simulink model "walkingRobotRL3D"  (R2020b)
settings: Solver=ode23t  StartTime=0.0  StopTime=Tf  RelTol=1e-2  EnableMultiTasking=on
PreLoadFcn:
  | robotParametersRL
undefined symbols (not defined in the file): agent, ankleD_pitch_jointMAX, ankleD_pitch_jointMIN, ankleD_roll_jointMAX, ankleD_roll_jointMIN, ankleI_pitch_jointMAX, ankleI_pitch_jointMIN, ankleI_roll_jointMAX, ankleI_roll_jointMIN, getSampleTime, height_plane, hipD_pitch_jointMAX, hipD_pitch_jointMIN, hipD_roll_jointMAX, hipD_roll_jointMIN, hipI_pitch_jointMAX, hipI_pitch_jointMIN, hipI_roll_jointMAX, hipI_roll_jointMIN, init_angs_L, init_angs_R, init_height, joint_damping, joint_limit_damping, joint_limit_stiffness, joint_stiffness, kneeD_jointMAX, kneeD_jointMIN, kneeI_jointMAX, kneeI_jointMIN, lower_leg_I0, lower_leg_length, lower_leg_mass, lower_leg_x, lower_leg_y, muscle_nominal_length, p10_ankleD_roll, plane_x, plane_y, regulator_type, tau, Tf, torso_height, torso_length, torso_offset_x, torso_offset_z, torso_width, torso_x, torso_y, torso_z, Ts, upper_leg_I0, upper_leg_length, upper_leg_mass, upper_leg_x, upper_leg_y, v10_ankleD_pitch, v10_ankleD_roll, v10_ankleI_pitch, v10_ankleI_roll ... (+41)
libraries: sm_lib x222, simulink x183, nesl_utility x130, walkingRobotUtils x69, rllib x2
(part 19 of 24)

== matlab function walkingRobotRL3D/Walking Robot/DYNAMIC MODEL OF PAM FOR LEFT LEG/Dynamic Model Antagonisitic PAM2/Proportional Regulator (Muscles 1) ==
  data: V1 input; reg_type input; p1 output
% Author: Eduardo Reyero Ibáñez
% Descrition: In this file it will be implemented the required input for the PAM
function p1  = propReg(V1,reg_type)
%% Proportional pressure regulators VPPM
%Range of Voltage
minVoltage = 0;
maxVoltage = 7.98; % This voltage provide 8 bar of pressure with regulator type 1
p1 = zeros(1,1);
%Select regulartor type
%reg_type = 1; % This will be given by the call of the function
%Limit the voltage
for i=1:length(p1)
if V1(i) >= maxVoltage 
    V1(i) = maxVoltage;
end
end
if reg_type == 1
    f_prop = @(V) 0.99*V+0.1;
    for i=1:length(p1)
    p1(i) = f_prop(V1(i));
    end
elseif reg_type == 2
    f_prop = @(V) 0.594*V+0.06;
    for i=1:length(p1)
    p1(i) = f_prop(V1(i));
    end
else
    f_prop = @(V) 0.198*V+0.02;
    for i=1:length(p1)
    p1(i) = f_prop(V1(i));
    end
end

% figure
% fplot(p1)
% xlim([0 10])
% ylim([0 10])
end

== matlab function walkingRobotRL3D/Walking Robot/DYNAMIC MODEL OF PAM FOR LEFT LEG/Dynamic Model Antagonisitic PAM2/Proportional Regulator (Muscles 2) ==
  data: V1 input; reg_type input; p1 output
% Author: Eduardo Reyero Ibáñez
% Descrition: In this file it will be implemented the required input for the PAM
function p1  = propReg(V1,reg_type)
%% Proportional pressure regulators VPPM
%Range of Voltage
minVoltage = 0;
maxVoltage = 7.98; % This voltage provide 8 bar of pressure with regulator type 1
p1 = zeros(1,1);
%Select regulartor type
%reg_type = 1; % This will be given by the call of the function
%Limit the voltage
for i=1:length(p1)
if V1(i) >= maxVoltage 
    V1(i) = maxVoltage;
end
end
if reg_type == 1
    f_prop = @(V) 0.99*V+0.1;
    for i=1:length(p1)
    p1(i) = f_prop(V1(i));
    end
elseif reg_type == 2
    f_prop = @(V) 0.594*V+0.06;
    for i=1:length(p1)
    p1(i) = f_prop(V1(i));
    end
else
    f_prop = @(V) 0.198*V+0.02;
    for i=1:length(p1)
    p1(i) = f_prop(V1(i));
    end
end

% figure
% fplot(p1)
% xlim([0 10])
% ylim([0 10])
end

== matlab function walkingRobotRL3D/Walking Robot/DYNAMIC MODEL OF PAM FOR LEFT LEG/Dynamic Model Antagonisitic PAM2/Spring and damping model/S(P),D(P) ==
  data: P1 input; S1 output; P2 input; D1 output; S2 output; D2 output
function [S1,D1,S2,D2] = getSpringDampingCoeff(P1,P2)
tau = 0.6;
% Spring and damping coeff for muscle 1
if P1>=0 && P1<=1
    S1 = 400;
    D1 = tau*S1;
elseif P1>1 && P1<=2
    S1 = 500;
    D1 = tau*S1;
elseif P1>2 && P1<=3
    S1 = 1100;
    D1 = tau*S1;
elseif P1>3 && P1<=4
    S1 = 1500;
    D1 = tau*S1;
elseif P1>4 && P1<=5
    S1 = 2000;
    D1 = tau*S1;
elseif P1>5 && P1<=6
    S1 = 2900;
    D1 = tau*S1;
elseif P1>6 && P1<=7
    S1 = 3800;
    D1 = tau*S1;
elseif P1>7 && P1<=8.5
    S1 = 5000;
    D1 = tau*S1;
else %Never will enter here
    S1 = 800;
    D1 = tau*S1;  
end

% Spring and damping coeff for muscle 1
if P2>=0 && P2<=1
    S2 = 400;
    D2 = tau*S2;
elseif P2>1 && P2<=2
    S2 = 500;
    D2 = tau*S2;
elseif P2>2 && P2<=3
    S2 = 1100;
    D2 = tau*S2;
elseif P2>3 && P2<=4
    S2 = 1500;
    D2 = tau*S2;
elseif P2>4 && P2<=5
    S2 = 2000;
    D2 = tau*S2;
elseif P2>5 && P2<=6
    S2 = 2900;
    D2 = tau*S2;
elseif P2>6 && P2<=7
    S2 = 3800;
    D2 = tau*S2;
elseif P2>7 && P2<=8.5
    S2 = 5000;
    D2 = tau*S2;
else %Never will enter here
    S2 = 800;
    D2 = tau*S2;  
end

end

== matlab function walkingRobotRL3D/Walking Robot/DYNAMIC MODEL OF PAM FOR LEFT LEG/Dynamic Model Antagonisitic PAM3/F(x,P) mode (Muscles 1) ==
  data: P1 input; F1 output; x_muscle1 input
%Author: Eduardo Reyero Ibáñez
%Note: F(x) curves for different pressures are limited by recommended
%limitation of 20% in contraction percentage for the used PAM actuator
%(L = 260mm D=20mm)
function F1 = FxPmodel(P1,x_muscle1)
%Input: P comming from proporcional controller  is in bar. Its 6x1 vector
% x_muscle (in % contraction)
%Output:F according to P input and and x value of half of the maximun
%permissible stroke
%Importing 2 variable F(x,P) model
curve = @(x,P)  -0.002697-93.8*x+2.917*P+13.05*x^2-0.04264*x*P-0.001793*P^2-0.9395*x^3-0.001597*x^2*P-0.0001142*x*P^2+4.694e-06*P^3+0.03335*x^4+6.106e-06*x^3*P+2.699e-06*x^2*P^2+1.25e-07*x*P^3-5.675e-09*P^4-0.0004611*x^5+9.334e-07*x^4*P-1.221e-08*x^3*P^2-1.463e-09*x^2*P^3-4.929e-11*x*P^4+2.492e-12*P^5;
%Defining F and x vectors for the 6 actuators
F1 = zeros(length(P1),1); %6x1
x1 = zeros(length(P1),1); %6x1
% Transform P from bar to Kpa
P1 = 100*P1;

for i=1:length(P1)
% Obtaining the stroke
x1(i) = x_muscle1(i); 
% Obtaining the applied force
F1(i) = curve(x1(i),P1(i)); 
if F1(i)<0
    F1(i) = 0;
end
end
end

== matlab function walkingRobotRL3D/Walking Robot/DYNAMIC MODEL OF PAM FOR LEFT LEG/Dynamic Model Antagonisitic PAM3/F(x,P) mode (Muscles 1)1 ==
  data: P2 input; F2 output; x_muscle2 input
%Author: Eduardo Reyero Ibáñez
%Note: F(x) curves for different pressures are limited by recommended
%limitation of 20% in contraction percentage for the used PAM actuator
%(L = 260mm D=20mm)
function F2 = FxPmodel(P2,x_muscle2)
%Input: P comming from proporcional controller  is in bar. Its 6x1 vector
% x_muscle (in % contraction)
%Output:F according to P input and and x value of half of the maximun
%permissible stroke
%Importing 2 variable F(x,P) model
curve = @(x,P)  -0.002697-93.8*x+2.917*P+13.05*x^2-0.04264*x*P-0.001793*P^2-0.9395*x^3-0.001597*x^2*P-0.0001142*x*P^2+4.694e-06*P^3+0.03335*x^4+6.106e-06*x^3*P+2.699e-06*x^2*P^2+1.25e-07*x*P^3-5.675e-09*P^4-0.0004611*x^5+9.334e-07*x^4*P-1.221e-08*x^3*P^2-1.463e-09*x^2*P^3-4.929e-11*x*P^4+2.492e-12*P^5;
%Defining F and x vectors for the 6 actuators
F2 = zeros(length(P2),1); %6x1
x2 = zeros(length(P2),1); %6x1
% Transform P from bar to Kpa
P2 = 100*P2;

for i=1:length(P2)
% Obtaining the stroke
x2(i) = x_muscle2(i); 
% Obtaining the applied force
F2(i) = curve(x2(i),P2(i));
if F2(i)<0
    F2(i) = 0;
end
end
end

== matlab function walkingRobotRL3D/Walking Robot1/Dynamic model of antagonistic PAM actuators/F(x,P) mode (Muscles 1) ==
  data: P1 input; F1 output; x_muscle1 input
%Author: Eduardo Reyero Ibáñez
%Note: F(x) curves for different pressures are limited by recommended
%limitation of 20% in contraction percentage for the used PAM actuator
%(L = 260mm D=20mm)
function F1 = FxPmodel(P1,x_muscle1)
%Input: P comming from proporcional controller  is in bar. Its 6x1 vector
% x_muscle (in % contraction)
%Output:F according to P input and and x value of half of the maximun
%permissible stroke
%Importing 2 variable F(x,P) model
curve = @(x,P)  -0.002697-93.8*x+2.917*P+13.05*x^2-0.04264*x*P-0.001793*P^2-0.9395*x^3-0.001597*x^2*P-0.0001142*x*P^2+4.694e-06*P^3+0.03335*x^4+6.106e-06*x^3*P+2.699e-06*x^2*P^2+1.25e-07*x*P^3-5.675e-09*P^4-0.0004611*x^5+9.334e-07*x^4*P-1.221e-08*x^3*P^2-1.463e-09*x^2*P^3-4.929e-11*x*P^4+2.492e-12*P^5;
%Defining F and x vectors for the 6 actuators
F1 = zeros(length(P1),1); %6x1
x1 = zeros(length(P1),1); %6x1
% Transform P from bar to Kpa
P1 = 100*P1;

for i=1:length(P1)
% Obtaining the stroke
x1(i) = x_muscle1(i); 
% Obtaining the applied force
F1(i) = curve(x1(i),P1(i)); 
end
end

== matlab function walkingRobotRL3D/Walking Robot/DYNAMIC MODEL OF PAM FOR LEFT LEG/Dynamic Model Antagonisitic PAM3/Proportional Regulator (Muscles 1) ==
  data: V1 input; reg_type input; p1 output
% Author: Eduardo Reyero Ibáñez
% Descrition: In this file it will be implemented the required input for the PAM
function p1  = propReg(V1,reg_type)
%% Proportional pressure regulators VPPM
%Range of Voltage
minVoltage = 0;
maxVoltage = 7.98; % This voltage provide 8 bar of pressure with regulator type 1
p1 = zeros(1,1);
%Select regulartor type
%reg_type = 1; % This will be given by the call of the function
%Limit the voltage
for i=1:length(p1)
if V1(i) >= maxVoltage 
    V1(i) = maxVoltage;
end
end
if reg_type == 1
    f_prop = @(V) 0.99*V+0.1;
    for i=1:length(p1)
    p1(i) = f_prop(V1(i));
    end
elseif reg_type == 2
    f_prop = @(V) 0.594*V+0.06;
    for i=1:length(p1)
    p1(i) = f_prop(V1(i));
    end
else
    f_prop = @(V) 0.198*V+0.02;
    for i=1:length(p1)
    p1(i) = f_prop(V1(i));
    end
end

% figure
% fplot(p1)
% xlim([0 10])
% ylim([0 10])
end

== matlab function walkingRobotRL3D/Walking Robot/DYNAMIC MODEL OF PAM FOR LEFT LEG/Dynamic Model Antagonisitic PAM3/Proportional Regulator (Muscles 2) ==
  data: V1 input; reg_type input; p1 output
% Author: Eduardo Reyero Ibáñez
% Descrition: In this file it will be implemented the required input for the PAM
function p1  = propReg(V1,reg_type)
%% Proportional pressure regulators VPPM
%Range of Voltage
minVoltage = 0;
maxVoltage = 7.98; % This voltage provide 8 bar of pressure with regulator type 1
p1 = zeros(1,1);
%Select regulartor type
%reg_type = 1; % This will be given by the call of the function
%Limit the voltage
for i=1:length(p1)
if V1(i) >= maxVoltage 
    V1(i) = maxVoltage;
end
end
if reg_type == 1
    f_prop = @(V) 0.99*V+0.1;
    for i=1:length(p1)
    p1(i) = f_prop(V1(i));
    end
elseif reg_type == 2
    f_prop = @(V) 0.594*V+0.06;
    for i=1:length(p1)
    p1(i) = f_prop(V1(i));
    end
else
    f_prop = @(V) 0.198*V+0.02;
    for i=1:length(p1)
    p1(i) = f_prop(V1(i));
    end
end

% figure
% fplot(p1)
% xlim([0 10])
% ylim([0 10])
end

== matlab function walkingRobotRL3D/Walking Robot/DYNAMIC MODEL OF PAM FOR LEFT LEG/Dynamic Model Antagonisitic PAM3/Spring and damping model/S(P),D(P) ==
  data: P1 input; S1 output; P2 input; D1 output; S2 output; D2 output
function [S1,D1,S2,D2] = getSpringDampingCoeff(P1,P2)
tau = 0.6;
% Spring and damping coeff for muscle 1
if P1>=0 && P1<=1
    S1 = 400;
    D1 = tau*S1;
elseif P1>1 && P1<=2
    S1 = 500;
    D1 = tau*S1;
elseif P1>2 && P1<=3
    S1 = 1100;
    D1 = tau*S1;
elseif P1>3 && P1<=4
    S1 = 1500;
    D1 = tau*S1;
elseif P1>4 && P1<=5
    S1 = 2000;
    D1 = tau*S1;
elseif P1>5 && P1<=6
    S1 = 2900;
    D1 = tau*S1;
elseif P1>6 && P1<=7
    S1 = 3800;
    D1 = tau*S1;
elseif P1>7 && P1<=8.5
    S1 = 5000;
    D1 = tau*S1;
else %Never will enter here
    S1 = 800;
    D1 = tau*S1;  
end

% Spring and damping coeff for muscle 1
if P2>=0 && P2<=1
    S2 = 400;
    D2 = tau*S2;
elseif P2>1 && P2<=2
    S2 = 500;
    D2 = tau*S2;
elseif P2>2 && P2<=3
    S2 = 1100;
    D2 = tau*S2;
elseif P2>3 && P2<=4
    S2 = 1500;
    D2 = tau*S2;
elseif P2>4 && P2<=5
    S2 = 2000;
    D2 = tau*S2;
elseif P2>5 && P2<=6
    S2 = 2900;
    D2 = tau*S2;
elseif P2>6 && P2<=7
    S2 = 3800;
    D2 = tau*S2;
elseif P2>7 && P2<=8.5
    S2 = 5000;
    D2 = tau*S2;
else %Never will enter here
    S2 = 800;
    D2 = tau*S2;  
end

end

== matlab function walkingRobotRL3D/Walking Robot1/Dynamic model of antagonistic PAM actuators/Spring//Damping (Muscles 2)/Getxmax2/getMaxStroke2 ==
  data: P2 input; x_max2 output
%Author: Eduardo Reyero Ibáñez
%Description: Functions for obtaining the maximun stroke value of a given
%curve F(x). It is reached for the x value which makes F = 0
function x_max2 = getMaxStroke(P2)
x_range = (-3:0.01:29)'; %This range convers the %contraction for all the pressures from 0 to 8 bar
%load('StaticFxPmodel\fxpSurface.mat');
curve1 = @(x,P)  -0.002697-93.8*x+2.917*P+13.05*x^2-0.04264*x*P-0.001793*P^2-0.9395*x^3-0.001597*x^2*P-0.0001142*x*P^2+4.694e-06*P^3+0.03335*x^4+6.106e-06*x^3*P+2.699e-06*x^2*P^2+1.25e-07*x*P^3-5.675e-09*P^4-0.0004611*x^5+9.334e-07*x^4*P-1.221e-08*x^3*P^2-1.463e-09*x^2*P^3-4.929e-11*x*P^4+2.492e-12*P^5;
F_x = zeros(length(x_range),1);
for i=1:length(x_range)
    F_x(i) = curve1(x_range(i),P2);
    if F_x(i)<0
       %We have found the x axis cross
       x_max2 = x_range(i-1);
       break;
   else
        x_max2 = x_range(i); %Will never end here but need to avoid simulink error
    end
end

end

== matlab function walkingRobotRL3D/Walking Robot/DYNAMIC MODEL OF PAM FOR LEFT LEG/Dynamic Model Antagonisitic PAM4/F(x,P) mode (Muscles 1) ==
  data: P1 input; F1 output; x_muscle1 input
%Author: Eduardo Reyero Ibáñez
%Note: F(x) curves for different pressures are limited by recommended
%limitation of 20% in contraction percentage for the used PAM actuator
%(L = 260mm D=20mm)
function F1 = FxPmodel(P1,x_muscle1)
%Input: P comming from proporcional controller  is in bar. Its 6x1 vector
% x_muscle (in % contraction)
%Output:F according to P input and and x value of half of the maximun
%permissible stroke
%Importing 2 variable F(x,P) model
curve = @(x,P)  -0.002697-93.8*x+2.917*P+13.05*x^2-0.04264*x*P-0.001793*P^2-0.9395*x^3-0.001597*x^2*P-0.0001142*x*P^2+4.694e-06*P^3+0.03335*x^4+6.106e-06*x^3*P+2.699e-06*x^2*P^2+1.25e-07*x*P^3-5.675e-09*P^4-0.0004611*x^5+9.334e-07*x^4*P-1.221e-08*x^3*P^2-1.463e-09*x^2*P^3-4.929e-11*x*P^4+2.492e-12*P^5;
%Defining F and x vectors for the 6 actuators
F1 = zeros(length(P1),1); %6x1
x1 = zeros(length(P1),1); %6x1
% Transform P from bar to Kpa
P1 = 100*P1;

for i=1:length(P1)
% Obtaining the stroke
x1(i) = x_muscle1(i); 
% Obtaining the applied force
F1(i) = curve(x1(i),P1(i)); 
if F1(i)<0
    F1(i) = 0;
end
end
end

== matlab function walkingRobotRL3D/Action+CI3/MATLAB Function ==
  data: x1 input; v1 output; v2 output
function [v1,v2]=ankleD_action(x1)
v1_values = [1.6809 1.72]';
v2_values = [1.6807 1.64]';
v1 = v1_values(1);
v2 = v2_values(1);
if  x1(1)>=14.05 
    v1 = v1_values(2);
    v2 = v2_values(2);
end
  
end

== matlab function walkingRobotRL3D/Walking Robot2/Dynamic model of antagonistic PAM actuators/F(x,P) mode (Muscles 1) ==
  data: P1 input; F1 output; x_muscle1 input
%Author: Eduardo Reyero Ibáñez
%Note: F(x) curves for different pressures are limited by recommended
%limitation of 20% in contraction percentage for the used PAM actuator
%(L = 260mm D=20mm)
function F1 = FxPmodel(P1,x_muscle1)
%Input: P comming from proporcional controller  is in bar. Its 6x1 vector
% x_muscle (in % contraction)
%Output:F according to P input and and x value of half of the maximun
%permissible stroke
%Importing 2 variable F(x,P) model
curve = @(x,P)  -0.002697-93.8*x+2.917*P+13.05*x^2-0.04264*x*P-0.001793*P^2-0.9395*x^3-0.001597*x^2*P-0.0001142*x*P^2+4.694e-06*P^3+0.03335*x^4+6.106e-06*x^3*P+2.699e-06*x^2*P^2+1.25e-07*x*P^3-5.675e-09*P^4-0.0004611*x^5+9.334e-07*x^4*P-1.221e-08*x^3*P^2-1.463e-09*x^2*P^3-4.929e-11*x*P^4+2.492e-12*P^5;
%Defining F and x vectors for the 6 actuators
F1 = zeros(length(P1),1); %6x1
x1 = zeros(length(P1),1); %6x1
% Transform P from bar to Kpa
P1 = 100*P1;

for i=1:length(P1)
% Obtaining the stroke
x1(i) = x_muscle1(i); 
% Obtaining the applied force
F1(i) = curve(x1(i),P1(i)); 
end
end

== matlab function walkingRobotRL3D/Walking Robot2/Dynamic model of antagonistic PAM actuators/F(x,P) model1 (Muscles 2) ==
  data: P2 input; F2 output; x_muscle2 input
%Author: Eduardo Reyero Ibáñez
%Note: F(x) curves for different pressures are limited by recommended
%limitation of 20% in contraction percentage for the used PAM actuator
%(L = 260mm D=20mm)
function F2 = FxPmodel(P2,x_muscle2)
%Input: P comming from proporcional controller  is in bar. Its 6x1 vector
% x_muscle2 in (% contraction)
%Output:F according to P input and and x value of half of the maximun
%permissible stroke
%Importing 2 variable F(x,P) model
curve = @(x,P)  -0.002697-93.8*x+2.917*P+13.05*x^2-0.04264*x*P-0.001793*P^2-0.9395*x^3-0.001597*x^2*P-0.0001142*x*P^2+4.694e-06*P^3+0.03335*x^4+6.106e-06*x^3*P+2.699e-06*x^2*P^2+1.25e-07*x*P^3-5.675e-09*P^4-0.0004611*x^5+9.334e-07*x^4*P-1.221e-08*x^3*P^2-1.463e-09*x^2*P^3-4.929e-11*x*P^4+2.492e-12*P^5;

%Defining F and x vectors for the 6 actuators
F2 = zeros(length(P2),1); %6x1
x2 = zeros(length(P2),1); %6x1
%x2 = [14.06 28.12 14.06 14.06 28.12 14.06]';
% Transform P from bar to Kpa
P2 = 100*P2;

for i=1:length(P2)
% Obtaining the stroke max/2
x2(i) = x_muscle2(i); 
% Obtaining the applied force
F2(i) = curve(x2(i),P2(i)); 
end
end

== matlab function walkingRobotRL3D/Walking Robot2/Dynamic model of antagonistic PAM actuators/F-->Torque ==
  data: x1 input; q output; x2 input
%Author: Eduardo Reyero
%Description: This file provides the Torque to apply to each joint of the
%robot based on the F(x) model input
%Input: Two 10x1 matrix of Forces. First matrix has the F1 forces which
%apply one of the two muscles on each joint. F2 has the forces that applied
%the second muscle on each joint
%Output: 10x1 torque vector(one component for each joint)
function q = get_angles(x1,x2)
%Define function
q = zeros(length(x1),1);
%Defining radius of the pulleys (m) (define values when know them)
r_ankle_roll = 0.03;% NOTE: THE ANKLE DOES NOT HAVE THIS MECHANISM.. THINK VARIANT
r_knee = 0.05;
r_hip_roll = 0.05;
r_ankle_pitch = 0.03; % NOTE: THE ANKLE DOES NOT HAVE THIS MECHANISM.. THINK VARIANT
r_hip_pitch = 0.05;


%AnkleD_roll
x10_ankleD_roll = 14.06*0.26/100; % In (m)
x20_ankleD_roll = 14.05*0.26/100; % In (m)
q(1) =(abs(x1(1)-x10_ankleD_roll)+abs(x2(1)-x20_ankleD_roll))/r_ankle_roll;
if x1(1) >= x10_ankleD_roll
    q(1) = q(1);
else
    q(1) = - q(1);
end
if q(1) > 5*pi/36
    q(1) = 5*pi/36;
end
if q(1) < -7*pi/36
    q(1) = -7*pi/36;
end


%AnkleD_pitch
x10_ankleD_pitch = 14.06*0.26/100; % In (m)
x20_ankleD_pitch = 14.05*0.26/100; % In (m)
q(2) =(abs(x1(2)-x10_ankleD_pitch)+abs(x2(2)-x20_ankleD_pitch))/r_ankle_pitch;
if x1(2) >= x10_ankleD_pitch
    q(2) = q(2);
else
    q(2) = - q(2);
end
if q(2) > pi/4
    q(2) = pi/4;
end
if q(2) < -pi/4
    q(2) = -pi/4;
end

%KneeD
x10_kneeD = 0.32*0.26/100; 
x20_kneeD = 28.12*0.26/100;
q(3) =(abs(x1(3)-x10_kneeD)+abs(x2(3)-x20_kneeD))/r_knee; % Knee only moves backwards
if q(3) > pi/2
    q(3) = pi/2;
end
if q(3) < 0
    q(3) = 0;
end

%HipD_roll
x10_hipD_roll = 14.06*0.26/100; % In (m)
x20_hipD_roll = 14.05*0.26/100; % In (m)
q(4) =(abs(x1(4)-x10_hipD_roll)+abs(x2(4)-x20_hipD_roll))/r_hip_roll;
if x1(4) >= x10_hipD_roll
    q(4) = q(4);
else
    q(4) = - q(4);
end
if q(4) > pi/8
    q(4) = pi/8;
end
if q(4) < -pi/16
    q(4) = -pi/16;
end

%Hip D pitch
x10_hipD_pitch = 14.06*0.26/100; % In (m)
x20_hipD_pitch = 14.05*0.26/100; % In (m)
q(5) =(abs(x1(5)-x10_hipD_pitch)+abs(x2(5)-x20_hipD_pitch))/r_hip_pitch;
if x1(5) >= x10_hipD_pitch
    q(5) = q(5);
else
    q(5) = - q(5);
end
if q(5) > pi/6   %pi/4
    q(5) = pi/6;      %pi/4;
end
if q(5) < -pi/4
    q(5) = -pi/4;
end

%AnkleI_roll
x10_ankleI_roll = 14.06*0.26/100; % In (m)
x20_ankleI_roll = 14.05*0.26/100; % In (m)
q(6) =(abs(x1(6)-x10_ankleI_roll)+abs(x2(6)-x20_ankleI_roll))/r_ankle_roll;
if x1(6) >= x10_ankleI_roll
    q(6) = q(6);
else
    q(6) = - q(6);
end
if q(6) > 7*pi/36
    q(6) = 7*pi/36;
end
if q(6) < -5*pi/36
    q(6) = -5*pi/36;
end

%AnkleI_pitch
x10_ankleI_pitch = 14.06*0.26/100; % In (m)
x20_ankleI_pitch = 14.05*0.26/100; % In (m)
q(7) =(abs(x1(7)-x10_ankleI_pitch)+abs(x2(7)-x20_ankleI_pitch))/r_ankle_pitch;
if x1(7) >= x10_ankleI_pitch
    q(7) = q(7);
else
    q(7) = - q(7);
end
if q(7) > pi/4
    q(7) = pi/4;
end
if q(7) < -pi/4
    q(7) = -pi/4;
end

%KneeI

x10_kneeI = 0.32*0.26/100; 
x20_kneeI = 28.12*0.26/100;
q(8) =(abs(x1(8)-x10_kneeI)+abs(x2(8)-x20_kneeI))/r_knee; % Knee only moves backwards
if q(8) > pi/2
    q(8) = pi/2;
end
if q(8) < 0
    q(8) = 0;
end

%HipI_roll
x10_hipI_roll = 14.06*0.26/100; % In (m)
x20_hipI_roll = 14.05*0.26/100; % In (m)
q(9) =(abs(x1(9)-x10_hipI_roll)+abs(x2(9)-x20_hipI_roll))/r_hip_roll;
if x1(9) >= x10_hipI_roll
    q(9) = q(9);
else
    q(9) = - q(9);
end
if q(9) > pi/16
    q(9) = pi/16;
end
if q(9) < -pi/8
    q(9) = -pi/8;
end

%Hip I pitch
x10_hipI_pitch = 14.06*0.26/100; % In (m)
x20_hipI_pitch = 14.05*0.26/100; % In (m)
q(10) =(abs(x1(10)-x10_hipI_pitch)+abs(x2(10)-x20_hipI_pitch))/r_hip_pitch;
if x1(10) >= x10_hipI_pitch
    q(10) = q(10);
else
    q(10) = - q(10);
end
if q(10) > pi/6   %pi/4
    q(10) = pi/6;     %pi/4;
end
if q(10) < -pi/4
    q(10) = -pi/4;
end

end

== matlab function walkingRobotRL3D/Walking Robot2/Dynamic model of antagonistic PAM actuators/Proportional Regulator (Muscles 1) ==
  data: V1 input; reg_type input; p1 output
% Author: Eduardo Reyero Ibáñez
% Descrition: In this file it will be implemented the required input for the PAM
function p1  = propReg(V1,reg_type)
%% Proportional pressure regulators VPPM
%Range of Voltage
minVoltage = 0;
maxVoltage = 7.98; % This voltage provide 8 bar of pressure with regulator type 1
p1 = zeros(10,1);
%Initial pressure for muscles
%p1 = [1.764 0 1.764 1.764 0 1.764]';

%Select regulartor type
%reg_type = 1; % This will be given by the call of the function
%Limit the voltage
for i=1:length(p1)
if V1(i) >= maxVoltage 
    V1(i) = maxVoltage;
end
end
if reg_type == 1
    f_prop = @(V) 0.99*V+0.1;
    for i=1:length(p1)
    p1(i) = f_prop(V1(i));
    end
elseif reg_type == 2
    f_prop = @(V) 0.594*V+0.06;
    for i=1:length(p1)
    p1(i) = f_prop(V1(i));
    end
else
    f_prop = @(V) 0.198*V+0.02;
    for i=1:length(p1)
    p1(i) = f_prop(V1(i));
    end
end

% figure
% fplot(p1)
% xlim([0 10])
% ylim([0 10])
end

== matlab function walkingRobotRL3D/Walking Robot2/Dynamic model of antagonistic PAM actuators/Proportional Regulator (Muscles 2) ==
  data: V2 input; p2 output; reg_type input
% Author: Eduardo Reyero Ibáñez
% Descrition: In this file it will be implemented the required input for the PAM
function p2 = propReg(V2,reg_type)
%% Proportional pressure regulators VPPM
%Range of Voltage
minVoltage = 0;
maxVoltage = 7.98; % This voltage provide 8 bar of pressure with regulator type 1
p2 = zeros(10,1);
%Initial pressure for muscles
%p2 = [1.764 8 1.764 1.764 8 1.764]';

%Select regulartor type
%reg_type = 1; % This will be given by the call of the function
%Limit the voltage
for i=1:length(p2)
if V2(i) >= maxVoltage 
    V2(i) = maxVoltage;
end
end
if reg_type == 1
    f_prop = @(V) 0.99*V+0.1;
    for i=1:length(p2)
    p2(i) = f_prop(V2(i));
    end
elseif reg_type == 2
    f_prop = @(V) 0.594*V+0.06;
    for i=1:length(p2)
    p2(i) = f_prop(V2(i));
    end
else
    f_prop = @(V) 0.198*V+0.02;
    for i=1:length(p2)
    p2(i) = f_prop(V2(i));
    end
end

% figure
% fplot(p2)
% xlim([0 10])
% ylim([0 10])
end

== matlab function walkingRobotRL3D/Walking Robot2/Dynamic model of antagonistic PAM actuators/Spring//Damping (Muscles 1)/Getxmax1/getMaxStroke ==
  data: P1 input; x_max1 output
%Author: Eduardo Reyero Ibáñez
%Description: Functions for obtaining the maximun stroke value of a given
%curve F(x). It is reached for the x value which makes F = 0
function x_max1 = getMaxStroke(P1)
x_range = (-3:0.01:29)'; %This range convers the %contraction for all the pressures from 0 to 8 bar
%load('StaticFxPmodel\fxpSurface.mat');
curve1 = @(x,P)  -0.002697-93.8*x+2.917*P+13.05*x^2-0.04264*x*P-0.001793*P^2-0.9395*x^3-0.001597*x^2*P-0.0001142*x*P^2+4.694e-06*P^3+0.03335*x^4+6.106e-06*x^3*P+2.699e-06*x^2*P^2+1.25e-07*x*P^3-5.675e-09*P^4-0.0004611*x^5+9.334e-07*x^4*P-1.221e-08*x^3*P^2-1.463e-09*x^2*P^3-4.929e-11*x*P^4+2.492e-12*P^5;
F_x = zeros(length(x_range),1);
for i=1:length(x_range)
    F_x(i) = curve1(x_range(i),P1);
    if F_x(i)<0
       %We have found the x axis cross
       x_max1 = x_range(i-1);
       break;
   else
        x_max1 = x_range(i); %Will never end here but need to avoid simulink error
    end
end

end

== matlab function walkingRobotRL3D/Walking Robot1/Dynamic model of antagonistic PAM actuators/Spring//Damping (Muscles 2)/Getxmax2/getMaxStroke3 ==
  data: P2 input; x_max2 output
%Author: Eduardo Reyero Ibáñez
%Description: Functions for obtaining the maximun stroke value of a given
%curve F(x). It is reached for the x value which makes F = 0
function x_max2 = getMaxStroke(P2)
x_range = (-3:0.01:29)'; %This range convers the %contraction for all the pressures from 0 to 8 bar
%load('StaticFxPmodel\fxpSurface.mat');
curve1 = @(x,P)  -0.002697-93.8*x+2.917*P+13.05*x^2-0.04264*x*P-0.001793*P^2-0.9395*x^3-0.001597*x^2*P-0.0001142*x*P^2+4.694e-06*P^3+0.03335*x^4+6.106e-06*x^3*P+2.699e-06*x^2*P^2+1.25e-07*x*P^3-5.675e-09*P^4-0.0004611*x^5+9.334e-07*x^4*P-1.221e-08*x^3*P^2-1.463e-09*x^2*P^3-4.929e-11*x*P^4+2.492e-12*P^5;
F_x = zeros(length(x_range),1);
for i=1:length(x_range)
    F_x(i) = curve1(x_range(i),P2);
    if F_x(i)<0
       %We have found the x axis cross
       x_max2 = x_range(i-1);
       break;
   else
        x_max2 = x_range(i); %Will never end here but need to avoid simulink error
    end
end

end

== matlab function walkingRobotRL3D/Walking Robot2/Dynamic model of antagonistic PAM actuators/Spring//Damping (Muscles 1)/Getxmax1/getMaxStroke1 ==
  data: P1 input; x_max1 output
%Author: Eduardo Reyero Ibáñez
%Description: Functions for obtaining the maximun stroke value of a given
%curve F(x). It is reached for the x value which makes F = 0
function x_max1 = getMaxStroke(P1)
x_range = (-3:0.01:29)'; %This range convers the %contraction for all the pressures from 0 to 8 bar
%load('StaticFxPmodel\fxpSurface.mat');
curve1 = @(x,P)  -0.002697-93.8*x+2.917*P+13.05*x^2-0.04264*x*P-0.001793*P^2-0.9395*x^3-0.001597*x^2*P-0.0001142*x*P^2+4.694e-06*P^3+0.03335*x^4+6.106e-06*x^3*P+2.699e-06*x^2*P^2+1.25e-07*x*P^3-5.675e-09*P^4-0.0004611*x^5+9.334e-07*x^4*P-1.221e-08*x^3*P^2-1.463e-09*x^2*P^3-4.929e-11*x*P^4+2.492e-12*P^5;
F_x = zeros(length(x_range),1);
for i=1:length(x_range)
    F_x(i) = curve1(x_range(i),P1);
    if F_x(i)<0
       %We have found the x axis cross
       x_max1 = x_range(i-1);
       break;
    else
        x_max1 = x_range(i); %Will never end here but need to avoid simulink error
    end
end

end

== matlab function walkingRobotRL3D/Walking Robot2/Dynamic model of antagonistic PAM actuators/Spring//Damping (Muscles 1)/Getxmax1/getMaxStroke2 ==
  data: P1 input; x_max1 output
%Author: Eduardo Reyero Ibáñez
%Description: Functions for obtaining the maximun stroke value of a given
%curve F(x). It is reached for the x value which makes F = 0
function x_max1 = getMaxStroke(P1)
x_range = (-3:0.01:29)'; %This range convers the %contraction for all the pressures from 0 to 8 bar
%load('StaticFxPmodel\fxpSurface.mat');
curve1 = @(x,P)  -0.002697-93.8*x+2.917*P+13.05*x^2-0.04264*x*P-0.001793*P^2-0.9395*x^3-0.001597*x^2*P-0.0001142*x*P^2+4.694e-06*P^3+0.03335*x^4+6.106e-06*x^3*P+2.699e-06*x^2*P^2+1.25e-07*x*P^3-5.675e-09*P^4-0.0004611*x^5+9.334e-07*x^4*P-1.221e-08*x^3*P^2-1.463e-09*x^2*P^3-4.929e-11*x*P^4+2.492e-12*P^5;
F_x = zeros(length(x_range),1);
for i=1:length(x_range)
    F_x(i) = curve1(x_range(i),P1);
    if F_x(i)<0
       %We have found the x axis cross
       x_max1 = x_range(i-1);
       break;
   else
        x_max1 = x_range(i); %Will never end here but need to avoid simulink error
    end
end

end

== matlab function walkingRobotRL3D/Walking Robot2/Dynamic model of antagonistic PAM actuators/Spring//Damping (Muscles 1)/Getxmax1/getMaxStroke3 ==
  data: P1 input; x_max1 output
%Author: Eduardo Reyero Ibáñez
%Description: Functions for obtaining the maximun stroke value of a given
%curve F(x). It is reached for the x value which makes F = 0
function x_max1 = getMaxStroke(P1)
x_range = (-3:0.01:29)'; %This range convers the %contraction for all the pressures from 0 to 8 bar
%load('StaticFxPmodel\fxpSurface.mat');
curve1 = @(x,P)  -0.002697-93.8*x+2.917*P+13.05*x^2-0.04264*x*P-0.001793*P^2-0.9395*x^3-0.001597*x^2*P-0.0001142*x*P^2+4.694e-06*P^3+0.03335*x^4+6.106e-06*x^3*P+2.699e-06*x^2*P^2+1.25e-07*x*P^3-5.675e-09*P^4-0.0004611*x^5+9.334e-07*x^4*P-1.221e-08*x^3*P^2-1.463e-09*x^2*P^3-4.929e-11*x*P^4+2.492e-12*P^5;
F_x = zeros(length(x_range),1);
for i=1:length(x_range)
    F_x(i) = curve1(x_range(i),P1);
    if F_x(i)<0
       %We have found the x axis cross
       x_max1 = x_range(i-1);
       break;
   else
        x_max1 = x_range(i); %Will never end here but need to avoid simulink error
    end
end

end

== matlab function walkingRobotRL3D/Walking Robot2/Dynamic model of antagonistic PAM actuators/Spring//Damping (Muscles 1)/Getxmax1/getMaxStroke4 ==
  data: P1 input; x_max1 output
%Author: Eduardo Reyero Ibáñez
%Description: Functions for obtaining the maximun stroke value of a given
%curve F(x). It is reached for the x value which makes F = 0
function x_max1 = getMaxStroke(P1)
x_range = (-3:0.01:29)'; %This range convers the %contraction for all the pressures from 0 to 8 bar
%load('StaticFxPmodel\fxpSurface.mat');
curve1 = @(x,P)  -0.002697-93.8*x+2.917*P+13.05*x^2-0.04264*x*P-0.001793*P^2-0.9395*x^3-0.001597*x^2*P-0.0001142*x*P^2+4.694e-06*P^3+0.03335*x^4+6.106e-06*x^3*P+2.699e-06*x^2*P^2+1.25e-07*x*P^3-5.675e-09*P^4-0.0004611*x^5+9.334e-07*x^4*P-1.221e-08*x^3*P^2-1.463e-09*x^2*P^3-4.929e-11*x*P^4+2.492e-12*P^5;
F_x = zeros(length(x_range),1);
for i=1:length(x_range)
    F_x(i) = curve1(x_range(i),P1);
    if F_x(i)<0
       %We have found the x axis cross
       x_max1 = x_range(i-1);
       break;
   else
        x_max1 = x_range(i); %Will never end here but need to avoid simulink error
    end
end

end

== matlab function walkingRobotRL3D/Walking Robot2/Dynamic model of antagonistic PAM actuators/Spring//Damping (Muscles 1)/Getxmax1/getMaxStroke5 ==
  data: P1 input; x_max1 output
%Author: Eduardo Reyero Ibáñez
%Description: Functions for obtaining the maximun stroke value of a given
%curve F(x). It is reached for the x value which makes F = 0
function x_max1 = getMaxStroke(P1)
x_range = (-3:0.01:29)'; %This range convers the %contraction for all the pressures from 0 to 8 bar
%load('StaticFxPmodel\fxpSurface.mat');
curve1 = @(x,P)  -0.002697-93.8*x+2.917*P+13.05*x^2-0.04264*x*P-0.001793*P^2-0.9395*x^3-0.001597*x^2*P-0.0001142*x*P^2+4.694e-06*P^3+0.03335*x^4+6.106e-06*x^3*P+2.699e-06*x^2*P^2+1.25e-07*x*P^3-5.675e-09*P^4-0.0004611*x^5+9.334e-07*x^4*P-1.221e-08*x^3*P^2-1.463e-09*x^2*P^3-4.929e-11*x*P^4+2.492e-12*P^5;
F_x = zeros(length(x_range),1);
for i=1:length(x_range)
    F_x(i) = curve1(x_range(i),P1);
    if F_x(i)<0
       %We have found the x axis cross
       x_max1 = x_range(i-1);
       break;
   else
        x_max1 = x_range(i); %Will never end here but need to avoid simulink error
    end
end

end

== matlab function walkingRobotRL3D/Walking Robot2/Dynamic model of antagonistic PAM actuators/Spring//Damping (Muscles 1)/Getxmax1/getMaxStroke6 ==
  data: P1 input; x_max1 output
%Author: Eduardo Reyero Ibáñez
%Description: Functions for obtaining the maximun stroke value of a given
%curve F(x). It is reached for the x value which makes F = 0
function x_max1 = getMaxStroke(P1)
x_range = (-3:0.01:29)'; %This range convers the %contraction for all the pressures from 0 to 8 bar
%load('StaticFxPmodel\fxpSurface.mat');
curve1 = @(x,P)  -0.002697-93.8*x+2.917*P+13.05*x^2-0.04264*x*P-0.001793*P^2-0.9395*x^3-0.001597*x^2*P-0.0001142*x*P^2+4.694e-06*P^3+0.03335*x^4+6.106e-06*x^3*P+2.699e-06*x^2*P^2+1.25e-07*x*P^3-5.675e-09*P^4-0.0004611*x^5+9.334e-07*x^4*P-1.221e-08*x^3*P^2-1.463e-09*x^2*P^3-4.929e-11*x*P^4+2.492e-12*P^5;
F_x = zeros(length(x_range),1);
for i=1:length(x_range)
    F_x(i) = curve1(x_range(i),P1);
    if F_x(i)<0
       %We have found the x axis cross
       x_max1 = x_range(i-1);
       break;
   else
        x_max1 = x_range(i); %Will never end here but need to avoid simulink error
    end
end

end

== matlab function walkingRobotRL3D/Walking Robot2/Dynamic model of antagonistic PAM actuators/Spring//Damping (Muscles 1)/Getxmax1/getMaxStroke7 ==
  data: P1 input; x_max1 output
%Author: Eduardo Reyero Ibáñez
%Description: Functions for obtaining the maximun stroke value of a given
%curve F(x). It is reached for the x value which makes F = 0
function x_max1 = getMaxStroke(P1)
x_range = (-3:0.01:29)'; %This range convers the %contraction for all the pressures from 0 to 8 bar
%load('StaticFxPmodel\fxpSurface.mat');
curve1 = @(x,P)  -0.002697-93.8*x+2.917*P+13.05*x^2-0.04264*x*P-0.001793*P^2-0.9395*x^3-0.001597*x^2*P-0.0001142*x*P^2+4.694e-06*P^3+0.03335*x^4+6.106e-06*x^3*P+2.699e-06*x^2*P^2+1.25e-07*x*P^3-5.675e-09*P^4-0.0004611*x^5+9.334e-07*x^4*P-1.221e-08*x^3*P^2-1.463e-09*x^2*P^3-4.929e-11*x*P^4+2.492e-12*P^5;
F_x = zeros(length(x_range),1);
for i=1:length(x_range)
    F_x(i) = curve1(x_range(i),P1);
    if F_x(i)<0
       %We have found the x axis cross
       x_max1 = x_range(i-1);
       break;
   else
        x_max1 = x_range(i); %Will never end here but need to avoid simulink error
    end
end

end

== matlab function walkingRobotRL3D/Walking Robot2/Dynamic model of antagonistic PAM actuators/Spring//Damping (Muscles 1)/Getxmax1/getMaxStroke8 ==
  data: P1 input; x_max1 output
%Author: Eduardo Reyero Ibáñez
%Description: Functions for obtaining the maximun stroke value of a given
%curve F(x). It is reached for the x value which makes F = 0
function x_max1 = getMaxStroke(P1)
x_range = (-3:0.01:29)'; %This range convers the %contraction for all the pressures from 0 to 8 bar
%load('StaticFxPmodel\fxpSurface.mat');
curve1 = @(x,P)  -0.002697-93.8*x+2.917*P+13.05*x^2-0.04264*x*P-0.001793*P^2-0.9395*x^3-0.001597*x^2*P-0.0001142*x*P^2+4.694e-06*P^3+0.03335*x^4+6.106e-06*x^3*P+2.699e-06*x^2*P^2+1.25e-07*x*P^3-5.675e-09*P^4-0.0004611*x^5+9.334e-07*x^4*P-1.221e-08*x^3*P^2-1.463e-09*x^2*P^3-4.929e-11*x*P^4+2.492e-12*P^5;
F_x = zeros(length(x_range),1);
for i=1:length(x_range)
    F_x(i) = curve1(x_range(i),P1);
    if F_x(i)<0
       %We have found the x axis cross
       x_max1 = x_range(i-1);
       break;
   else
        x_max1 = x_range(i); %Will never end here but need to avoid simulink error
    end
end

end

== matlab function walkingRobotRL3D/Walking Robot2/Dynamic model of antagonistic PAM actuators/Spring//Damping (Muscles 1)/Getxmax1/getMaxStroke9 ==
  data: P1 input; x_max1 output
%Author: Eduardo Reyero Ibáñez
%Description: Functions for obtaining the maximun stroke value of a given
%curve F(x). It is reached for the x value which makes F = 0
function x_max1 = getMaxStroke(P1)
x_range = (-3:0.01:29)'; %This range convers the %contraction for all the pressures from 0 to 8 bar
%load('StaticFxPmodel\fxpSurface.mat');
curve1 = @(x,P)  -0.002697-93.8*x+2.917*P+13.05*x^2-0.04264*x*P-0.001793*P^2-0.9395*x^3-0.001597*x^2*P-0.0001142*x*P^2+4.694e-06*P^3+0.03335*x^4+6.106e-06*x^3*P+2.699e-06*x^2*P^2+1.25e-07*x*P^3-5.675e-09*P^4-0.0004611*x^5+9.334e-07*x^4*P-1.221e-08*x^3*P^2-1.463e-09*x^2*P^3-4.929e-11*x*P^4+2.492e-12*P^5;
F_x = zeros(length(x_range),1);
for i=1:length(x_range)
    F_x(i) = curve1(x_range(i),P1);
    if F_x(i)<0
       %We have found the x axis cross
       x_max1 = x_range(i-1);
       break;
   else
        x_max1 = x_range(i); %Will never end here but need to avoid simulink error
    end
end

end

== matlab function walkingRobotRL3D/Walking Robot2/Dynamic model of antagonistic PAM actuators/Spring//Damping (Muscles 1)/MATLAB Function ==
  data: F1 input; S1 output; F2 input; xmax_muscles1 input
%Author: Eduardo Reyero
%Description: Calculate spring coefficient

function S1 = calculateSpringCoeff(F1,F2,xmax_muscles1)
S1=zeros(length(xmax_muscles1),1);
for i = 1:length(S1)
    S1(i) = (F1(i)-F2(i))/xmax_muscles1(i);
end

end

== matlab function walkingRobotRL3D/Walking Robot1/Dynamic model of antagonistic PAM actuators/Spring//Damping (Muscles 2)/Getxmax2/getMaxStroke4 ==
  data: P2 input; x_max2 output
%Author: Eduardo Reyero Ibáñez
%Description: Functions for obtaining the maximun stroke value of a given
%curve F(x). It is reached for the x value which makes F = 0
function x_max2 = getMaxStroke(P2)
x_range = (-3:0.01:29)'; %This range convers the %contraction for all the pressures from 0 to 8 bar
%load('StaticFxPmodel\fxpSurface.mat');
curve1 = @(x,P)  -0.002697-93.8*x+2.917*P+13.05*x^2-0.04264*x*P-0.001793*P^2-0.9395*x^3-0.001597*x^2*P-0.0001142*x*P^2+4.694e-06*P^3+0.03335*x^4+6.106e-06*x^3*P+2.699e-06*x^2*P^2+1.25e-07*x*P^3-5.675e-09*P^4-0.0004611*x^5+9.334e-07*x^4*P-1.221e-08*x^3*P^2-1.463e-09*x^2*P^3-4.929e-11*x*P^4+2.492e-12*P^5;
F_x = zeros(length(x_range),1);
for i=1:length(x_range)
    F_x(i) = curve1(x_range(i),P2);
    if F_x(i)<0
       %We have found the x axis cross
       x_max2 = x_range(i-1);
       break;
   else
        x_max2 = x_range(i); %Will never end here but need to avoid simulink error
    end
end

end

== matlab function walkingRobotRL3D/Walking Robot2/Dynamic model of antagonistic PAM actuators/Spring//Damping (Muscles 2)/Getxmax2/getMaxStroke ==
  data: P2 input; x_max2 output
%Author: Eduardo Reyero Ibáñez
%Description: Functions for obtaining the maximun stroke value of a given
%curve F(x). It is reached for the x value which makes F = 0
function x_max2 = getMaxStroke(P2)
x_range = (-3:0.01:29)'; %This range convers the %contraction for all the pressures from 0 to 8 bar
%load('StaticFxPmodel\fxpSurface.mat');
curve1 = @(x,P)  -0.002697-93.8*x+2.917*P+13.05*x^2-0.04264*x*P-0.001793*P^2-0.9395*x^3-0.001597*x^2*P-0.0001142*x*P^2+4.694e-06*P^3+0.03335*x^4+6.106e-06*x^3*P+2.699e-06*x^2*P^2+1.25e-07*x*P^3-5.675e-09*P^4-0.0004611*x^5+9.334e-07*x^4*P-1.221e-08*x^3*P^2-1.463e-09*x^2*P^3-4.929e-11*x*P^4+2.492e-12*P^5;
F_x = zeros(length(x_range),1);
for i=1:length(x_range)
    F_x(i) = curve1(x_range(i),P2);
    if F_x(i)<0
       %We have found the x axis cross
       x_max2 = x_range(i-1);
       break;
   else
        x_max2 = x_range(i); %Will never end here but need to avoid simulink error
    end
end

end

== matlab function walkingRobotRL3D/Walking Robot2/Dynamic model of antagonistic PAM actuators/Spring//Damping (Muscles 2)/Getxmax2/getMaxStroke1 ==
  data: P2 input; x_max2 output
%Author: Eduardo Reyero Ibáñez
%Description: Functions for obtaining the maximun stroke value of a given
%curve F(x). It is reached for the x value which makes F = 0
function x_max2 = getMaxStroke(P2)
x_range = (-3:0.01:29)'; %This range convers the %contraction for all the pressures from 0 to 8 bar
%load('StaticFxPmodel\fxpSurface.mat');
curve1 = @(x,P)  -0.002697-93.8*x+2.917*P+13.05*x^2-0.04264*x*P-0.001793*P^2-0.9395*x^3-0.001597*x^2*P-0.0001142*x*P^2+4.694e-06*P^3+0.03335*x^4+6.106e-06*x^3*P+2.699e-06*x^2*P^2+1.25e-07*x*P^3-5.675e-09*P^4-0.0004611*x^5+9.334e-07*x^4*P-1.221e-08*x^3*P^2-1.463e-09*x^2*P^3-4.929e-11*x*P^4+2.492e-12*P^5;
F_x = zeros(length(x_range),1);
for i=1:length(x_range)
    F_x(i) = curve1(x_range(i),P2);
    if F_x(i)<0
       %We have found the x axis cross
       x_max2 = x_range(i-1);
       break;
    else
        x_max2 = x_range(i); %Will never end here but need to avoid simulink error
    end
end

end

== matlab function walkingRobotRL3D/Walking Robot2/Dynamic model of antagonistic PAM actuators/Spring//Damping (Muscles 2)/Getxmax2/getMaxStroke2 ==
  data: P2 input; x_max2 output
%Author: Eduardo Reyero Ibáñez
%Description: Functions for obtaining the maximun stroke value of a given
%curve F(x). It is reached for the x value which makes F = 0
function x_max2 = getMaxStroke(P2)
x_range = (-3:0.01:29)'; %This range convers the %contraction for all the pressures from 0 to 8 bar
%load('StaticFxPmodel\fxpSurface.mat');
curve1 = @(x,P)  -0.002697-93.8*x+2.917*P+13.05*x^2-0.04264*x*P-0.001793*P^2-0.9395*x^3-0.001597*x^2*P-0.0001142*x*P^2+4.694e-06*P^3+0.03335*x^4+6.106e-06*x^3*P+2.699e-06*x^2*P^2+1.25e-07*x*P^3-5.675e-09*P^4-0.0004611*x^5+9.334e-07*x^4*P-1.221e-08*x^3*P^2-1.463e-09*x^2*P^3-4.929e-11*x*P^4+2.492e-12*P^5;
F_x = zeros(length(x_range),1);
for i=1:length(x_range)
    F_x(i) = curve1(x_range(i),P2);
    if F_x(i)<0
       %We have found the x axis cross
       x_max2 = x_range(i-1);
       break;
   else
        x_max2 = x_range(i); %Will never end here but need to avoid simulink error
    end
end

end

== matlab function walkingRobotRL3D/Walking Robot2/Dynamic model of antagonistic PAM actuators/Spring//Damping (Muscles 2)/Getxmax2/getMaxStroke3 ==
  data: P2 input; x_max2 output
%Author: Eduardo Reyero Ibáñez
%Description: Functions for obtaining the maximun stroke value of a given
%curve F(x). It is reached for the x value which makes F = 0
function x_max2 = getMaxStroke(P2)
x_range = (-3:0.01:29)'; %This range convers the %contraction for all the pressures from 0 to 8 bar
%load('StaticFxPmodel\fxpSurface.mat');
curve1 = @(x,P)  -0.002697-93.8*x+2.917*P+13.05*x^2-0.04264*x*P-0.001793*P^2-0.9395*x^3-0.001597*x^2*P-0.0001142*x*P^2+4.694e-06*P^3+0.03335*x^4+6.106e-06*x^3*P+2.699e-06*x^2*P^2+1.25e-07*x*P^3-5.675e-09*P^4-0.0004611*x^5+9.334e-07*x^4*P-1.221e-08*x^3*P^2-1.463e-09*x^2*P^3-4.929e-11*x*P^4+2.492e-12*P^5;
F_x = zeros(length(x_range),1);
for i=1:length(x_range)
    F_x(i) = curve1(x_range(i),P2);
    if F_x(i)<0
       %We have found the x axis cross
       x_max2 = x_range(i-1);
       break;
   else
        x_max2 = x_range(i); %Will never end here but need to avoid simulink error
    end
end

end

== matlab function walkingRobotRL3D/Walking Robot2/Dynamic model of antagonistic PAM actuators/Spring//Damping (Muscles 2)/Getxmax2/getMaxStroke4 ==
  data: P2 input; x_max2 output
%Author: Eduardo Reyero Ibáñez
%Description: Functions for obtaining the maximun stroke value of a given
%curve F(x). It is reached for the x value which makes F = 0
function x_max2 = getMaxStroke(P2)
x_range = (-3:0.01:29)'; %This range convers the %contraction for all the pressures from 0 to 8 bar
%load('StaticFxPmodel\fxpSurface.mat');
curve1 = @(x,P)  -0.002697-93.8*x+2.917*P+13.05*x^2-0.04264*x*P-0.001793*P^2-0.9395*x^3-0.001597*x^2*P-0.0001142*x*P^2+4.694e-06*P^3+0.03335*x^4+6.106e-06*x^3*P+2.699e-06*x^2*P^2+1.25e-07*x*P^3-5.675e-09*P^4-0.0004611*x^5+9.334e-07*x^4*P-1.221e-08*x^3*P^2-1.463e-09*x^2*P^3-4.929e-11*x*P^4+2.492e-12*P^5;
F_x = zeros(length(x_range),1);
for i=1:length(x_range)
    F_x(i) = curve1(x_range(i),P2);
    if F_x(i)<0
       %We have found the x axis cross
       x_max2 = x_range(i-1);
       break;
   else
        x_max2 = x_range(i); %Will never end here but need to avoid simulink error
    end
end

end

== matlab function walkingRobotRL3D/Walking Robot2/Dynamic model of antagonistic PAM actuators/Spring//Damping (Muscles 2)/Getxmax2/getMaxStroke5 ==
  data: P2 input; x_max2 output
%Author: Eduardo Reyero Ibáñez
%Description: Functions for obtaining the maximun stroke value of a given
%curve F(x). It is reached for the x value which makes F = 0
function x_max2 = getMaxStroke(P2)
x_range = (-3:0.01:29)'; %This range convers the %contraction for all the pressures from 0 to 8 bar
%load('StaticFxPmodel\fxpSurface.mat');
curve1 = @(x,P)  -0.002697-93.8*x+2.917*P+13.05*x^2-0.04264*x*P-0.001793*P^2-0.9395*x^3-0.001597*x^2*P-0.0001142*x*P^2+4.694e-06*P^3+0.03335*x^4+6.106e-06*x^3*P+2.699e-06*x^2*P^2+1.25e-07*x*P^3-5.675e-09*P^4-0.0004611*x^5+9.334e-07*x^4*P-1.221e-08*x^3*P^2-1.463e-09*x^2*P^3-4.929e-11*x*P^4+2.492e-12*P^5;
F_x = zeros(length(x_range),1);
for i=1:length(x_range)
    F_x(i) = curve1(x_range(i),P2);
    if F_x(i)<0
       %We have found the x axis cross
       x_max2 = x_range(i-1);
       break;
   else
        x_max2 = x_range(i); %Will never end here but need to avoid simulink error
    end
end

end

== matlab function walkingRobotRL3D/Walking Robot2/Dynamic model of antagonistic PAM actuators/Spring//Damping (Muscles 2)/Getxmax2/getMaxStroke6 ==
  data: P2 input; x_max2 output
%Author: Eduardo Reyero Ibáñez
%Description: Functions for obtaining the maximun stroke value of a given
%curve F(x). It is reached for the x value which makes F = 0
function x_max2 = getMaxStroke(P2)
x_range = (-3:0.01:29)'; %This range convers the %contraction for all the pressures from 0 to 8 bar
%load('StaticFxPmodel\fxpSurface.mat');
curve1 = @(x,P)  -0.002697-93.8*x+2.917*P+13.05*x^2-0.04264*x*P-0.001793*P^2-0.9395*x^3-0.001597*x^2*P-0.0001142*x*P^2+4.694e-06*P^3+0.03335*x^4+6.106e-06*x^3*P+2.699e-06*x^2*P^2+1.25e-07*x*P^3-5.675e-09*P^4-0.0004611*x^5+9.334e-07*x^4*P-1.221e-08*x^3*P^2-1.463e-09*x^2*P^3-4.929e-11*x*P^4+2.492e-12*P^5;
F_x = zeros(length(x_range),1);
for i=1:length(x_range)
    F_x(i) = curve1(x_range(i),P2);
    if F_x(i)<0
       %We have found the x axis cross
       x_max2 = x_range(i-1);
       break;
   else
        x_max2 = x_range(i); %Will never end here but need to avoid simulink error
    end
end

end

== matlab function walkingRobotRL3D/Walking Robot2/Dynamic model of antagonistic PAM actuators/Spring//Damping (Muscles 2)/Getxmax2/getMaxStroke7 ==
  data: P2 input; x_max2 output
%Author: Eduardo Reyero Ibáñez
%Description: Functions for obtaining the maximun stroke value of a given
%curve F(x). It is reached for the x value which makes F = 0
function x_max2 = getMaxStroke(P2)
x_range = (-3:0.01:29)'; %This range convers the %contraction for all the pressures from 0 to 8 bar
%load('StaticFxPmodel\fxpSurface.mat');
curve1 = @(x,P)  -0.002697-93.8*x+2.917*P+13.05*x^2-0.04264*x*P-0.001793*P^2-0.9395*x^3-0.001597*x^2*P-0.0001142*x*P^2+4.694e-06*P^3+0.03335*x^4+6.106e-06*x^3*P+2.699e-06*x^2*P^2+1.25e-07*x*P^3-5.675e-09*P^4-0.0004611*x^5+9.334e-07*x^4*P-1.221e-08*x^3*P^2-1.463e-09*x^2*P^3-4.929e-11*x*P^4+2.492e-12*P^5;
F_x = zeros(length(x_range),1);
for i=1:length(x_range)
    F_x(i) = curve1(x_range(i),P2);
    if F_x(i)<0
       %We have found the x axis cross
       x_max2 = x_range(i-1);
       break;
   else
        x_max2 = x_range(i); %Will never end here but need to avoid simulink error
    end
end

end

== matlab function walkingRobotRL3D/Walking Robot2/Dynamic model of antagonistic PAM actuators/Spring//Damping (Muscles 2)/Getxmax2/getMaxStroke8 ==
  data: P2 input; x_max2 output
%Author: Eduardo Reyero Ibáñez
%Description: Functions for obtaining the maximun stroke value of a given
%curve F(x). It is reached for the x value which makes F = 0
function x_max2 = getMaxStroke(P2)
x_range = (-3:0.01:29)'; %This range convers the %contraction for all the pressures from 0 to 8 bar
%load('StaticFxPmodel\fxpSurface.mat');
curve1 = @(x,P)  -0.002697-93.8*x+2.917*P+13.05*x^2-0.04264*x*P-0.001793*P^2-0.9395*x^3-0.001597*x^2*P-0.0001142*x*P^2+4.694e-06*P^3+0.03335*x^4+6.106e-06*x^3*P+2.699e-06*x^2*P^2+1.25e-07*x*P^3-5.675e-09*P^4-0.0004611*x^5+9.334e-07*x^4*P-1.221e-08*x^3*P^2-1.463e-09*x^2*P^3-4.929e-11*x*P^4+2.492e-12*P^5;
F_x = zeros(length(x_range),1);
for i=1:length(x_range)
    F_x(i) = curve1(x_range(i),P2);
    if F_x(i)<0
       %We have found the x axis cross
       x_max2 = x_range(i-1);
       break;
   else
        x_max2 = x_range(i); %Will never end here but need to avoid simulink error
    end
end

end

== matlab function walkingRobotRL3D/Walking Robot2/Dynamic model of antagonistic PAM actuators/Spring//Damping (Muscles 2)/Getxmax2/getMaxStroke9 ==
  data: P2 input; x_max2 output
%Author: Eduardo Reyero Ibáñez
%Description: Functions for obtaining the maximun stroke value of a given
%curve F(x). It is reached for the x value which makes F = 0
function x_max2 = getMaxStroke(P2)
x_range = (-3:0.01:29)'; %This range convers the %contraction for all the pressures from 0 to 8 bar
%load('StaticFxPmodel\fxpSurface.mat');
curve1 = @(x,P)  -0.002697-93.8*x+2.917*P+13.05*x^2-0.04264*x*P-0.001793*P^2-0.9395*x^3-0.001597*x^2*P-0.0001142*x*P^2+4.694e-06*P^3+0.03335*x^4+6.106e-06*x^3*P+2.699e-06*x^2*P^2+1.25e-07*x*P^3-5.675e-09*P^4-0.0004611*x^5+9.334e-07*x^4*P-1.221e-08*x^3*P^2-1.463e-09*x^2*P^3-4.929e-11*x*P^4+2.492e-12*P^5;
F_x = zeros(length(x_range),1);
for i=1:length(x_range)
    F_x(i) = curve1(x_range(i),P2);
    if F_x(i)<0
       %We have found the x axis cross
       x_max2 = x_range(i-1);
       break;
   else
        x_max2 = x_range(i); %Will never end here but need to avoid simulink error
    end
end

end

== matlab function walkingRobotRL3D/Walking Robot1/Dynamic model of antagonistic PAM actuators/Spring//Damping (Muscles 2)/Getxmax2/getMaxStroke5 ==
  data: P2 input; x_max2 output
%Author: Eduardo Reyero Ibáñez
%Description: Functions for obtaining the maximun stroke value of a given
%curve F(x). It is reached for the x value which makes F = 0
function x_max2 = getMaxStroke(P2)
x_range = (-3:0.01:29)'; %This range convers the %contraction for all the pressures from 0 to 8 bar
%load('StaticFxPmodel\fxpSurface.mat');
curve1 = @(x,P)  -0.002697-93.8*x+2.917*P+13.05*x^2-0.04264*x*P-0.001793*P^2-0.9395*x^3-0.001597*x^2*P-0.0001142*x*P^2+4.694e-06*P^3+0.03335*x^4+6.106e-06*x^3*P+2.699e-06*x^2*P^2+1.25e-07*x*P^3-5.675e-09*P^4-0.0004611*x^5+9.334e-07*x^4*P-1.221e-08*x^3*P^2-1.463e-09*x^2*P^3-4.929e-11*x*P^4+2.492e-12*P^5;
F_x = zeros(length(x_range),1);
for i=1:length(x_range)
    F_x(i) = curve1(x_range(i),P2);
    if F_x(i)<0
       %We have found the x axis cross
       x_max2 = x_range(i-1);
       break;
   else
        x_max2 = x_range(i); %Will never end here but need to avoid simulink error
    end
end

end
